simulink library "SENSORS"  (R2021b)
settings: Solver=VariableStepAuto  StartTime=0.0  StopTime=10.0  RelTol=1e-3
undefined symbols (not defined in the file or in its folder): alfaX, alfaXY, alfaXZ, alfaY, alfaYX, alfaYZ, alfaZ, alfaZX, alfaZY, angleSun, cMag, gaussian, h, hLens, Imax, maxStar, n, nLens, Nsens, stdDevMag, stdDevPhi, stdDevTheta
libraries: ERRORS x3, simulink x3, matrix_library x3, kinematic_transform x1
settings Model: Creator=Davide  LastModifiedBy=Davide

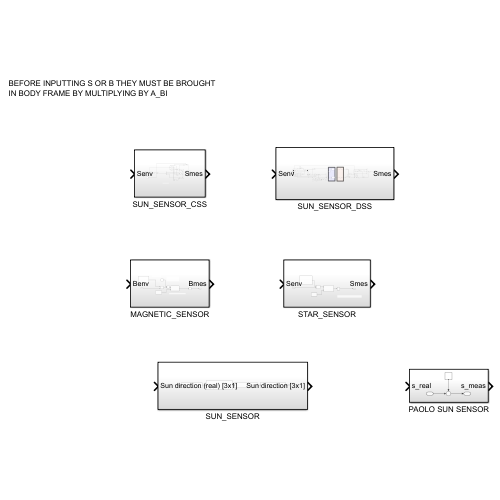
[thumbnail: Simulink's stored preview of the top-level diagram]
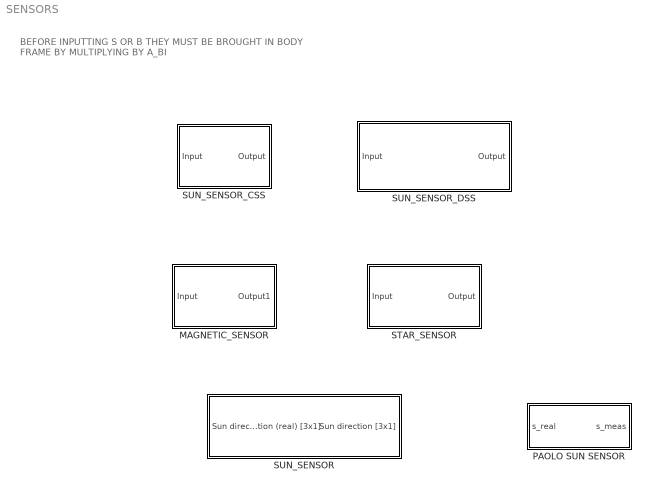
== system SENSORS ==
  note: BEFORE INPUTTING S OR B THEY MUST BE BROUGHT
      | IN BODY FRAME BY MULTIPLYING BY A_BI
  MAGNETIC_SENSOR : Subsystem
  PAOLO SUN SENSOR : Subsystem
  STAR_SENSOR : Subsystem
  SUN_SENSOR : Subsystem
  SUN_SENSOR_CSS : Subsystem
  SUN_SENSOR_DSS : Subsystem

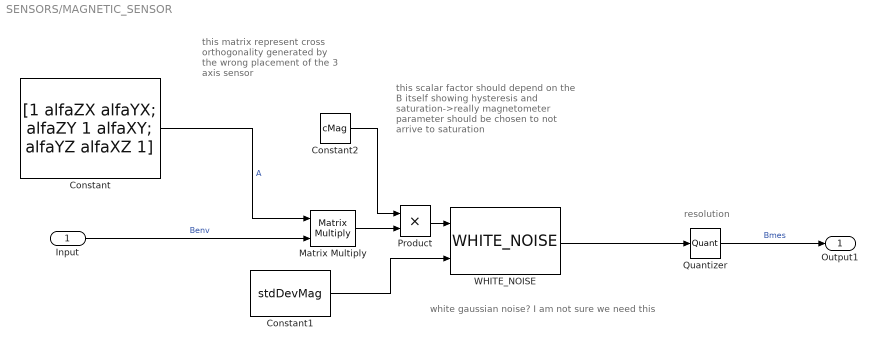
== system SENSORS/MAGNETIC_SENSOR ==
  note: resolution
  note: white gaussian noise? I am not sure we need this
  note: this scalar factor should depend
      | on the B itself showing hysteresis
      | and saturation->really magnetometer
      | parameter should be chosen to not
      | arrive to saturation
  note: this matrix represent cross
      | orthogonality generated
      | by the wrong placement of
      | the 3 axis sensor
  Input : Inport
  Constant : Constant  Value=[1 alfaZX alfaYX; alfaZY 1 alfaXY; alfaYZ alfaXZ 1]
  Constant1 : Constant  Value=stdDevMag
  Constant2 : Constant  Value=cMag
  Matrix Multiply : Product  Multiplication=Matrix(*)
  Product : Product
  Quantizer : Quantizer  QuantizationInterval=resMag
  WHITE_NOISE : ERRORS/WHITE_NOISE  SystemSampleTime=-1  VariantActivationTime=update diagram  Latency=0  AutoFrameSizeCalculation=off
      settings: SourceProductName=Errors
  Output1 : Outport
  wires:
  Input/1 -> Matrix Multiply/2  "Benv"
  Constant/1 -> Matrix Multiply/1  "A"
  Matrix Multiply/1 -> Product/2
  Constant1/1 -> WHITE_NOISE/2
  WHITE_NOISE/1 -> Quantizer/1
  Constant2/1 -> Product/1
  Product/1 -> WHITE_NOISE/1
  Quantizer/1 -> Output1/1  "Bmes"

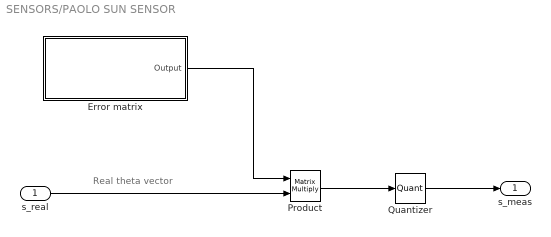
== system SENSORS/PAOLO SUN SENSOR ==
  note: Real theta vector
  s_real : Inport
  Error matrix : Subsystem
  Product : Product  Multiplication=Matrix(*)
  Quantizer : Quantizer  QuantizationInterval=resSun
  s_meas : Outport
  wires:
  s_real/1 -> Product/2
  Error matrix/1(Output) -> Product/1
  Product/1 -> Quantizer/1
  Quantizer/1 -> s_meas/1

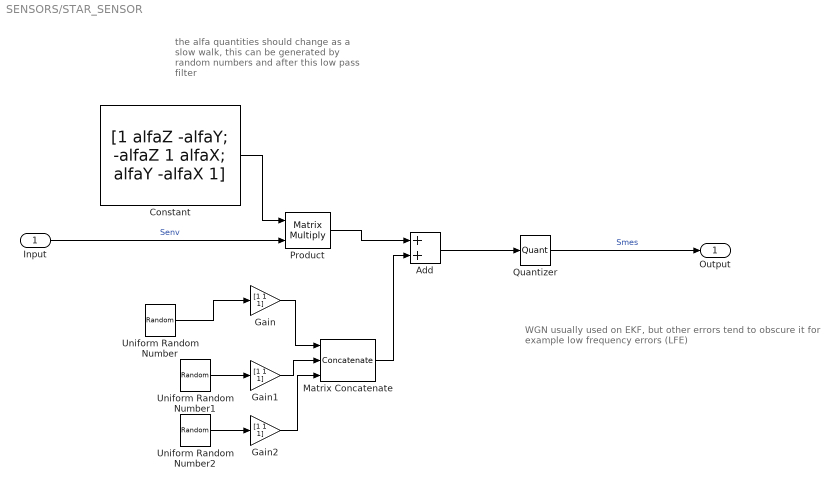
== system SENSORS/STAR_SENSOR ==
  note: the alfa quantities should change as
      | a slow walk, this can be generated by
      | random numbers and after this low
      | pass filter
  note: WGN usually used on EKF, but other errors tend to obscure it
      | for example low frequency errors (LFE)
  Input : Inport
  Add : Sum
  Constant : Constant  Value=[1 alfaZ -alfaY; -alfaZ 1 alfaX; alfaY -alfaX 1]
  Gain : Gain  Gain=[1 1 1]
  Gain1 : Gain  Gain=[1 1 1]
  Gain2 : Gain  Gain=[1 1 1]
  Matrix Concatenate : Concatenate  NumInputs=3  Mode=Multidimensional array  ConcatenateDimension=2
  Product : Product  Multiplication=Matrix(*)
  Quantizer : Quantizer  QuantizationInterval=resStar
  Uniform Random Number : UniformRandomNumber  Minimum=-maxStar  Maximum=maxStar  Seed=10  SampleTime=0.1
  Uniform Random Number1 : UniformRandomNumber  Minimum=-maxStar  Maximum=maxStar  Seed=8  SampleTime=0.1
  Uniform Random Number2 : UniformRandomNumber  Minimum=-maxStar  Maximum=maxStar  SampleTime=0.1
  Output : Outport
  wires:
  Quantizer/1 -> Output/1  "Smes"
  Input/1 -> Product/2  "Senv"
  Add/1 -> Quantizer/1
  Constant/1 -> Product/1
  Product/1 -> Add/1
  Uniform Random Number/1 -> Gain/1
  Uniform Random Number1/1 -> Gain1/1
  Uniform Random Number2/1 -> Gain2/1
  Gain1/1 -> Matrix Concatenate/2
  Gain2/1 -> Matrix Concatenate/3
  Gain/1 -> Matrix Concatenate/1
  Matrix Concatenate/1 -> Add/2

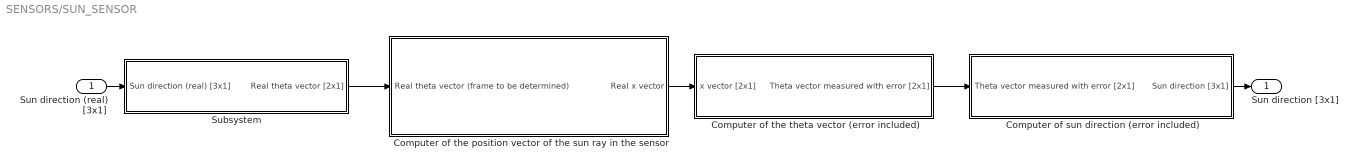
== system SENSORS/SUN_SENSOR ==
  Sun direction (real) [3x1] : Inport
  Computer of sun direction (error included) : Subsystem
  Computer of the position vector of the sun ray in the sensor : Subsystem
  Computer of the theta vector (error included) : Subsystem
  Subsystem : Subsystem
  Sun direction [3x1] : Outport
  wires:
  Subsystem/1(Real theta vector [2x1]) -> Computer of the position vector of the sun ray in the sensor/1(Real theta vector (frame to be determined))
  Computer of the position vector of the sun ray in the sensor/1(Real x vector) -> Computer of the theta vector (error included)/1(x vector [2x1])
  Computer of the theta vector (error included)/1(Theta vector measured with error [2x1]) -> Computer of sun direction (error included)/1(Theta vector measured with error [2x1])
  Computer of sun direction (error included)/1(Sun direction [3x1]) -> Sun direction [3x1]/1
  Sun direction (real) [3x1]/1 -> Subsystem/1(Sun direction (real) [3x1])

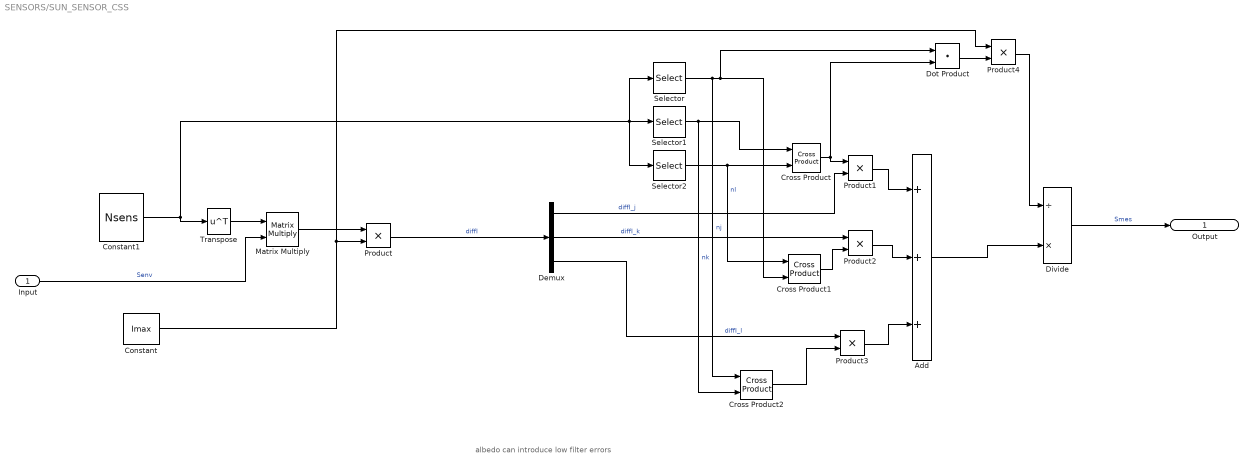
== system SENSORS/SUN_SENSOR_CSS ==
  note: albedo can introduce low filter errors
  Input : Inport
  Add : Sum  Inputs=+++
  Constant : Constant  Value=Imax
  Constant1 : Constant  Value=Nsens
  Cross Product : matrix_library/Cross Product
      settings: SourceProductBaseCode=SL
  Cross Product1 : matrix_library/Cross Product
      settings: SourceProductBaseCode=SL
  Cross Product2 : matrix_library/Cross Product
      settings: SourceProductBaseCode=SL
  Demux : Demux  Outputs=3
  Divide : Product  Inputs=/*
  Dot Product : DotProduct  InputSameDT=on  OutDataTypeStr=Inherit: Inherit via internal rule
  Matrix Multiply : Product  Multiplication=Matrix(*)
  Product{,1..4} (5 alike) : Product
  Selector : Selector  NumberOfDimensions=2  InputPortWidth=3  IndexOptions=Select all,Index vector (dialog)  Indices=1,1  OutputSizes=1,1
  Selector1 : Selector  NumberOfDimensions=2  InputPortWidth=3  IndexOptions=Select all,Index vector (dialog)  Indices=1,2  OutputSizes=1,1
  Selector2 : Selector  NumberOfDimensions=2  InputPortWidth=3  IndexOptions=Select all,Index vector (dialog)  Indices=1,3  OutputSizes=1,1
  Transpose : Math  Operator=transpose  SaturateOnIntegerOverflow=on
  Output : Outport
  wires:
  Selector1/1 -> Cross Product2/2, Cross Product/1  "nk"
  Constant1/1 -> Transpose/1, Selector2/1, Selector1/1, Selector/1
  Selector2/1 -> Cross Product1/1, Cross Product/2  "nl"
  Add/1 -> Divide/2
  Product3/1 -> Add/3
  Selector/1 -> Cross Product2/1, Dot Product/1, Cross Product1/2  "nj"
  Cross Product2/1 -> Product3/2
  Divide/1 -> Output/1  "Smes"
  Demux/1 -> Product1/2  "diffI_j"
  Matrix Multiply/1 -> Product/1
  Dot Product/1 -> Product4/2
  Constant/1 -> Product4/1, Product/2
  Product4/1 -> Divide/1
  Product/1 -> Demux/1  "diffI"
  Product2/1 -> Add/2
  Demux/2 -> Product2/1  "diffI_k"
  Product1/1 -> Add/1
  Cross Product/1 -> Dot Product/2, Product1/1
  Demux/3 -> Product3/1  "diffI_l"
  Cross Product1/1 -> Product2/2
  Input/1 -> Matrix Multiply/2  "Senv"
  Transpose/1 -> Matrix Multiply/1

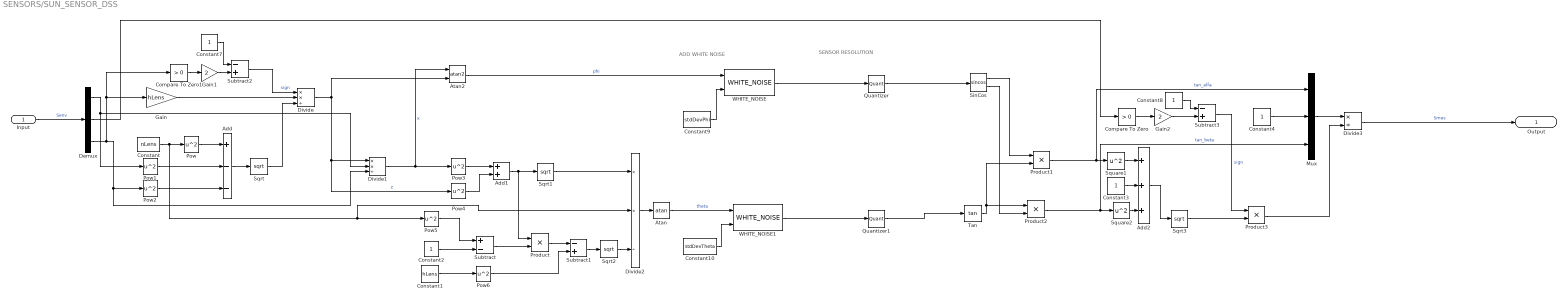
== system SENSORS/SUN_SENSOR_DSS ==
  note: SENSOR RESOLUTION
  note: ADD WHITE NOISE
  Input : Inport
  Add : Sum  Inputs=+--
  Add1 : Sum
  Add2 : Sum  Inputs=+++
  Atan : Trigonometry  Operator=atan
  Atan2 : Trigonometry  Operator=atan2
  Compare To Zero : simulink/Logic and Bit Operations/Compare To Zero  relop=>  OutDataTypeStr=boolean
  Compare To Zero1 : simulink/Logic and Bit Operations/Compare To Zero  relop=>  OutDataTypeStr=boolean
  Constant : Constant  Value=nLens
  Constant1 : Constant  Value=hLens
  Constant10 : Constant  Value=stdDevTheta
  Constant{2..4,7..8} (5 alike) : Constant
  Constant9 : Constant  Value=stdDevPhi
  Demux : Demux  Outputs=3
  Divide : Product  Inputs=**/
  Divide1 : Product  Inputs=**/
  Divide2 : Product  Inputs=**/
  Divide3 : Product  Inputs=*/
  Gain : Gain  Gain=hLens
  Gain1 : Gain  Gain=2
  Gain2 : Gain  Gain=2
  Mux : Mux  Inputs=3
  Pow{,1..6} (7 alike) : Math  Operator=square  SignedPower=on  RndMeth=Zero  SaturateOnIntegerOverflow=on
  Product{,1..3} (4 alike) : Product
  Quantizer : Quantizer  QuantizationInterval=resPhi
  Quantizer1 : Quantizer  QuantizationInterval=resTheta
  SinCos : Trigonometry  Operator=sincos
  Sqrt{,1..3} (4 alike) : Sqrt  SaturateOnIntegerOverflow=on
  Square1 : Math  Operator=square  SaturateOnIntegerOverflow=on
  Square2 : Math  Operator=square  SaturateOnIntegerOverflow=on
  Subtract : Sum  Inputs=+-
  Subtract1 : Sum  Inputs=-+
  Subtract2 : Sum  Inputs=-+
  Subtract3 : Sum  Inputs=-+
  Tan : Trigonometry  Operator=tan
  WHITE_NOISE : ERRORS/WHITE_NOISE  SystemSampleTime=-1  VariantActivationTime=update diagram  Latency=0  AutoFrameSizeCalculation=off
      settings: SourceProductName=Errors
  WHITE_NOISE1 : ERRORS/WHITE_NOISE  SystemSampleTime=-1  VariantActivationTime=update diagram  Latency=0  AutoFrameSizeCalculation=off
      settings: SourceProductName=Errors
  Output : Outport
  wires:
  Constant4/1 -> Mux/2
  Sqrt2/1 -> Divide2/3
  Product2/1 -> Square2/1, Mux/3  "tan_beta"
  Input/1 -> Demux/1  "Senv"
  Tan/1 -> Product1/2, Product2/1
  Divide1/1 -> Atan2/1, Pow3/1  "x"
  Mux/1 -> Divide3/1
  Pow4/1 -> Add1/2
  Add/1 -> Sqrt/1
  SinCos/1 -> Product1/1
  Add1/1 -> Product/1, Sqrt1/1
  Quantizer1/1 -> Tan/1
  Quantizer/1 -> SinCos/1
  Pow/1 -> Add/1
  Divide2/1 -> Atan/1
  SinCos/2 -> Product2/2
  Constant3/1 -> Add2/2
  Sqrt3/1 -> Product3/2
  Product/1 -> Subtract1/1
  Constant/1 -> Pow/1, Divide2/2, Pow5/1
  Demux/1 -> Pow1/1, Divide1/2
  Subtract1/1 -> Sqrt2/1
  Pow2/1 -> Add/3
  Product3/1 -> Divide3/2
  Add2/1 -> Sqrt3/1
  Pow5/1 -> Subtract/1
  Subtract/1 -> Product/2
  Pow6/1 -> Subtract1/2
  Divide/1 -> Atan2/2, Pow4/1, Divide1/1  "z"
  Pow1/1 -> Add/2
  Demux/3 -> Compare To Zero1/1, Gain/1, Pow2/1, Divide1/3
  Sqrt/1 -> Divide/3
  Gain/1 -> Divide/2
  Constant1/1 -> Pow6/1
  WHITE_NOISE1/1 -> Quantizer1/1
  Compare To Zero1/1 -> Gain1/1
  Demux/2 -> Compare To Zero/1
  Pow3/1 -> Add1/1
  Atan2/1 -> WHITE_NOISE/1  "phi"
  Compare To Zero/1 -> Gain2/1
  Product1/1 -> Square1/1, Mux/1  "tan_alfa"
  Sqrt1/1 -> Divide2/1
  Divide3/1 -> Output/1  "Smes"
  Atan/1 -> WHITE_NOISE1/1  "theta"
  Constant2/1 -> Subtract/2
  WHITE_NOISE/1 -> Quantizer/1
  Gain1/1 -> Subtract2/2
  Constant7/1 -> Subtract2/1
  Subtract2/1 -> Divide/1  "sign"
  Constant8/1 -> Subtract3/1
  Gain2/1 -> Subtract3/2
  Subtract3/1 -> Product3/1  "sign"
  Constant9/1 -> WHITE_NOISE/2
  Constant10/1 -> WHITE_NOISE1/2
  Square1/1 -> Add2/1
  Square2/1 -> Add2/3

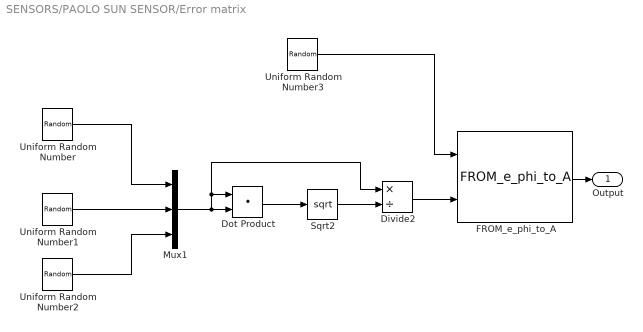
== system SENSORS/PAOLO SUN SENSOR/Error matrix ==
  Divide2 : Product  Inputs=*/
  Dot Product : DotProduct  InputSameDT=on  OutDataTypeStr=Inherit: Inherit via internal rule
  FROM_e_phi_to_A : kinematic_transform/FROM_e_phi_to_A  SystemSampleTime=-1  VariantActivationTime=update diagram  Latency=0  AutoFrameSizeCalculation=off
  Mux1 : Mux  Inputs=3
  Sqrt2 : Sqrt  SaturateOnIntegerOverflow=on
  Uniform Random Number : UniformRandomNumber  Minimum=-10  Maximum=10  Seed=1  SampleTime=0.1
  Uniform Random Number1 : UniformRandomNumber  Minimum=-10  Maximum=10  Seed=2  SampleTime=0.1
  Uniform Random Number2 : UniformRandomNumber  Minimum=-10  Maximum=10  Seed=3  SampleTime=0.1
  Uniform Random Number3 : UniformRandomNumber  Minimum=-angleSun  Maximum=angleSun  Seed=10  SampleTime=0.1
  Output : Outport
  wires:
  Sqrt2/1 -> Divide2/2
  Mux1/1 -> Dot Product/1, Divide2/1, Dot Product/2
  Uniform Random Number2/1 -> Mux1/3
  Divide2/1 -> FROM_e_phi_to_A/2
  Dot Product/1 -> Sqrt2/1
  Uniform Random Number/1 -> Mux1/1
  Uniform Random Number3/1 -> FROM_e_phi_to_A/1
  Uniform Random Number1/1 -> Mux1/2
  FROM_e_phi_to_A/1 -> Output/1

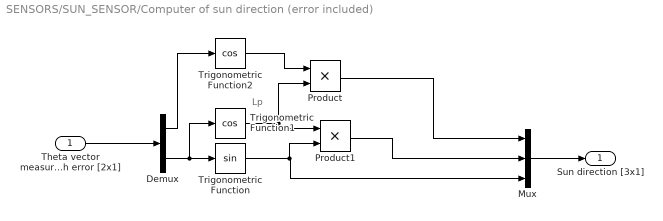
== system SENSORS/SUN_SENSOR/Computer of sun direction (error included) ==
  note: Lp
  Theta vector measured with error [2x1] : Inport
  Demux : Demux  Outputs=2
  Mux : Mux  Inputs=3
  Product : Product
  Product1 : Product
  Trigonometric Function : Trigonometry
  Trigonometric Function1 : Trigonometry  Operator=cos
  Trigonometric Function2 : Trigonometry  Operator=cos
  Sun direction [3x1] : Outport
  wires:
  Mux/1 -> Sun direction [3x1]/1
  Trigonometric Function2/1 -> Product/1
  Product1/1 -> Mux/2
  Trigonometric Function/1 -> Product1/2, Mux/3
  Trigonometric Function1/1 -> Product1/1, Product/2
  Demux/2 -> Trigonometric Function1/1, Trigonometric Function/1
  Demux/1 -> Trigonometric Function2/1
  Theta vector measured with error [2x1]/1 -> Demux/1
  Product/1 -> Mux/1

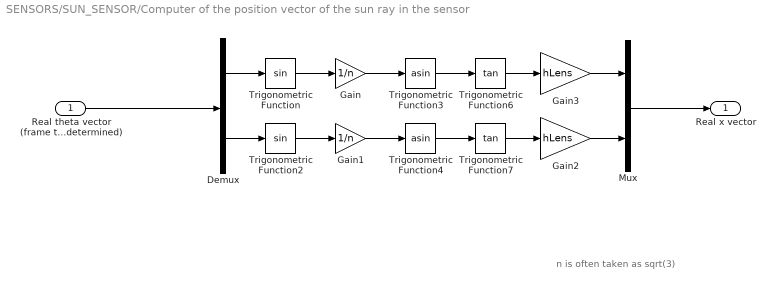
== system SENSORS/SUN_SENSOR/Computer of the position vector of the sun ray in the sensor ==
  note: n is often taken as sqrt(3)
  Real theta vector (frame to be determined) : Inport
  Demux : Demux  Outputs=2
  Gain : Gain  Gain=1/n
  Gain1 : Gain  Gain=1/n
  Gain2 : Gain  Gain=hLens
  Gain3 : Gain  Gain=hLens
  Mux : Mux  Inputs=2
  Trigonometric Function : Trigonometry
  Trigonometric Function2 : Trigonometry
  Trigonometric Function3 : Trigonometry  Operator=asin
  Trigonometric Function4 : Trigonometry  Operator=asin
  Trigonometric Function6 : Trigonometry  Operator=tan
  Trigonometric Function7 : Trigonometry  Operator=tan
  Real x vector : Outport
  wires:
  Demux/2 -> Trigonometric Function2/1
  Real theta vector (frame to be determined)/1 -> Demux/1
  Gain/1 -> Trigonometric Function3/1
  Trigonometric Function2/1 -> Gain1/1
  Mux/1 -> Real x vector/1
  Trigonometric Function7/1 -> Gain2/1
  Demux/1 -> Trigonometric Function/1
  Trigonometric Function/1 -> Gain/1
  Trigonometric Function3/1 -> Trigonometric Function6/1
  Trigonometric Function6/1 -> Gain3/1
  Trigonometric Function4/1 -> Trigonometric Function7/1
  Gain1/1 -> Trigonometric Function4/1
  Gain3/1 -> Mux/1
  Gain2/1 -> Mux/2

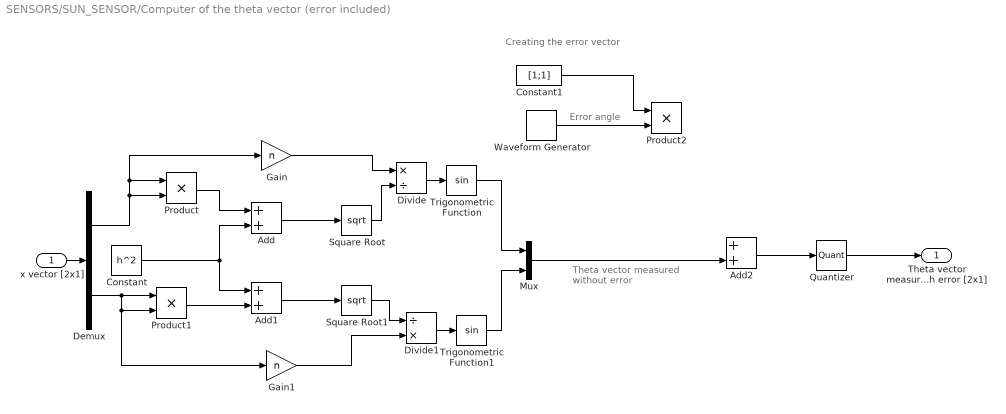
== system SENSORS/SUN_SENSOR/Computer of the theta vector (error included) ==
  note: Creating the error vector
  note: Theta vector measured
      |  without error
  note: Error angle
  x vector [2x1] : Inport
  Add : Sum
  Add1 : Sum
  Add2 : Sum
  Constant : Constant  Value=h^2
  Constant1 : Constant  Value=[1;1]
  Demux : Demux  Outputs=2
  Divide : Product  Inputs=*/
  Divide1 : Product  Inputs=/*
  Gain : Gain  Gain=n
  Gain1 : Gain  Gain=n
  Mux : Mux  Inputs=2
  Product : Product
  Product1 : Product
  Product2 : Product
  Quantizer : Quantizer  QuantizationInterval=res
  Square Root : Sqrt  SaturateOnIntegerOverflow=on
  Square Root1 : Sqrt  SaturateOnIntegerOverflow=on
  Trigonometric Function : Trigonometry
  Trigonometric Function1 : Trigonometry
  Waveform Generator : simulink/Sources/Waveform Generator  OutMin=[]  OutMax=[]  OutDataTypeStr=double  SelectedSignal=1  Signals=gaussian(0,0.01,6)  BlockNames=MultiportSwitch_1b8e21e75e6d46c  SampleTime=0.1
  Theta vector measured with error [2x1] : Outport
  wires:
  x vector [2x1]/1 -> Demux/1
  Add1/1 -> Square Root1/1
  Product/1 -> Add/1
  Trigonometric Function/1 -> Mux/1
  Mux/1 -> Add2/2
  Demux/1 -> Gain/1, Product/1, Product/2
  Divide/1 -> Trigonometric Function/1
  Add/1 -> Square Root/1
  Trigonometric Function1/1 -> Mux/2
  Square Root/1 -> Divide/2
  Demux/2 -> Gain1/1, Product1/2, Product1/1
  Constant/1 -> Add1/1, Add/2
  Gain/1 -> Divide/1
  Gain1/1 -> Divide1/2
  Divide1/1 -> Trigonometric Function1/1
  Product1/1 -> Add1/2
  Square Root1/1 -> Divide1/1
  Waveform Generator/1 -> Product2/2
  Constant1/1 -> Product2/1
  Add2/1 -> Quantizer/1
  Quantizer/1 -> Theta vector measured with error [2x1]/1

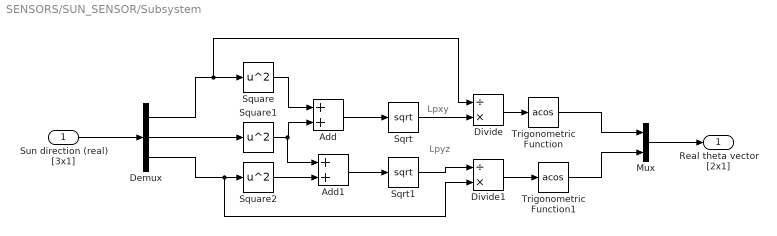
== system SENSORS/SUN_SENSOR/Subsystem ==
  note: Lpyz
  note: Lpxy
  Sun direction (real) [3x1] : Inport
  Add : Sum
  Add1 : Sum
  Demux : Demux  Outputs=3
  Divide : Product  Inputs=/*
  Divide1 : Product  Inputs=/*
  Mux : Mux  Inputs=2
  Sqrt : Sqrt  SaturateOnIntegerOverflow=on
  Sqrt1 : Sqrt  SaturateOnIntegerOverflow=on
  Square : Math  Operator=square  SaturateOnIntegerOverflow=on
  Square1 : Math  Operator=square  SaturateOnIntegerOverflow=on
  Square2 : Math  Operator=square  SaturateOnIntegerOverflow=on
  Trigonometric Function : Trigonometry  Operator=acos
  Trigonometric Function1 : Trigonometry  Operator=acos
  Real theta vector [2x1] : Outport
  wires:
  Demux/1 -> Divide/1, Square/1
  Trigonometric Function/1 -> Mux/1
  Square2/1 -> Add1/2
  Square1/1 -> Add1/1, Add/2
  Demux/2 -> Square1/1
  Divide/1 -> Trigonometric Function/1
  Trigonometric Function1/1 -> Mux/2
  Sun direction (real) [3x1]/1 -> Demux/1
  Sqrt/1 -> Divide/2
  Square/1 -> Add/1
  Demux/3 -> Divide1/2, Square2/1
  Add1/1 -> Sqrt1/1
  Sqrt1/1 -> Divide1/1
  Add/1 -> Sqrt/1
  Divide1/1 -> Trigonometric Function1/1
  Mux/1 -> Real theta vector [2x1]/1
